simulink model "DCM_Pulse_Converter_Compare"  (R2019a)
settings: Solver=ode5  StartTime=0.0  StopTime=t_end  FixedStep=dt  RelTol=1e-3  EnableMultiTasking=on
values from neighbouring files (symbols this model uses):
  dt = 1e-5    (= 1e-05)    [Experiment_1_DCM_Parameter.m]
  T_c = 0    [Experiment_1_DCM_Parameter.m]
  T_CON = 0    [Experiment_1_DCM_Parameter.m]
  U_EN = 220    [Experiment_1_DCM_Parameter.m]
  V_CON = 0    [Experiment_1_DCM_Parameter.m]
libraries: simulink x1, powerlib x1
settings Model: Creator=BinLi  LastModifiedBy=Praktikum
settings DataIOCC: LimitDataPoints=on  SaveFormat=Array  SignalLoggingSaveFormat=ModelDataLogs  ReturnWorkspaceOutputs=off
settings OptimizationCC: ExpressionDepthLimit=2147483647  LifeSpan=inf
settings DebuggingCC: UnderspecifiedInitializationDetection=Classic  MergeDetectMultiDrivingBlocksExec=none  SolverPrmCheckMsg=warning  FcnCallInpInsideContextMsg=warning  StateNameClashWarn=warning  SFUnexpectedBacktrackingDiag=warning  SFNoUnconditionalDefaultTransitionDiag=warning  SFExecutionAtInitializationDiag=none  ArithmeticOperatorsInVariantConditions=warning
settings HardwareCC: ProdBitPerPointer=32  ProdBitPerSizeT=32  ProdBitPerPtrDiffT=32  ProdLargestAtomicFloat=None  ProdIntDivRoundTo=Undefined  ProdEndianess=Unspecified  ProdWordSize=32  ProdHWDeviceType=32-bit Generic
settings ModelReferenceCC: PropagateSignalLabelsOutOfModel=off
settings SFSimCC: SimUseLocalCustomCode=off  SimParseCustomCode=off
settings RTWCC: RTWUseLocalCustomCode=off
settings CodeAppCC: StateflowObjectComments=on
settings GRTTargetCC: TargetLangStandard=C89/C90 (ANSI)  CombineOutputUpdateFcns=off  GRTInterface=on
settings ConfigComp: CovMetricSettings=dw  CovSaveCumulativeToWorkspaceVar=on  CovSaveSingleToWorkspaceVar=on  CovExternalEMLEnable=off  CovSFcnEnable=off
settings SimscapeCC: SimscapeNormalizeSystem=off

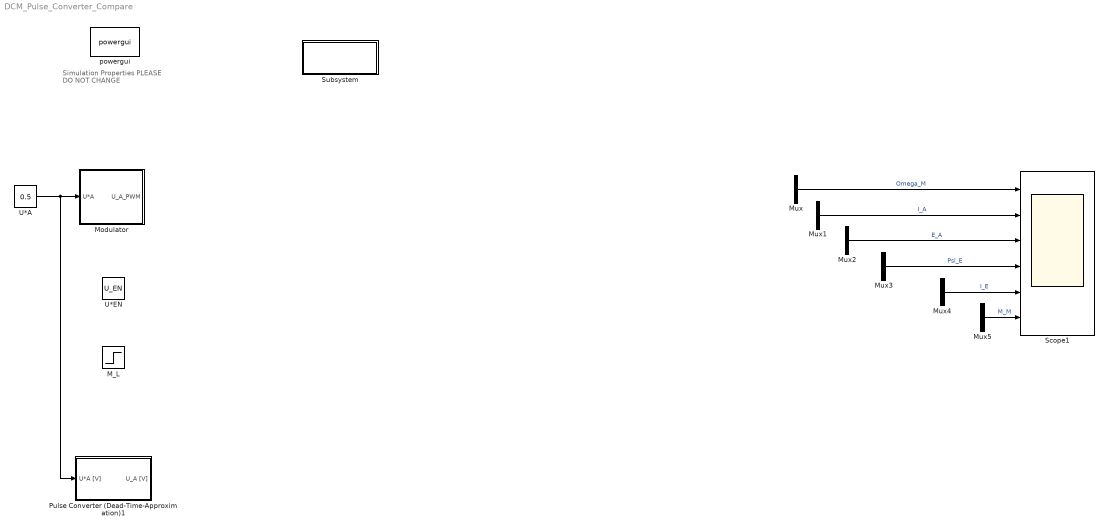
== system DCM_Pulse_Converter_Compare ==
  note: Simulation Properties
      | PLEASE DO NOT CHANGE
  M_L : Step  After=0.5  SampleTime=0
  Modulator : Subsystem
  Mux{,1..5} (6 alike) : Mux  Inputs=2
  Pulse Converter (Dead-Time-Approximation)1 : Subsystem
  Scope1 : Scope  NumInputPorts=6
  Subsystem : Subsystem
      settings: OpenFcn=Experiment_1_DCM_Parameter
      mask Display: disp('Initialize\n (doppelklicken)')
  U*A : Constant  Value=0.5
  U*EN : Constant  Value=U_EN
  powergui : powerlib/powergui  Priority=1  SimulationMode=Discrete  SampleTime=dt  frequency=60  Iterations=50  frequencyindice=0  Pbase=100e6  ErrMax=1e-4  UnitsV=kV  UnitsW=MW  buscounter=0  FunctionMessages=off  echomessages=off  EnableUseOfTLC=off  CurrentSourceSwitches=off  DisableSnubberDevices=off  DisableRonSwitches=off  DisableVfSwitches=off  DisplayEquations=off  AutomaticDiscreteSolvers=off  SolverType=Tustin  Interpol=off  ExternalGateDelay=off  methode=off  Ts=0  x0status=blocks  SPID=off  SwTol=0  HookPort=off  NonlinearTolerance=1e-4  nMaxIteration=100  ContinueOnMaxIteration=off  RestoreLinks=warning  ResistiveCurrentMeasurement=off  Frange=[0:2:500]  Ylog=off  Xlog=on  ShowGrid=off  save=off  variable=ZData  structure=0  ZoomFFT=off  StartTime=0.0  cycles=1  DisplayStyle=1  fundamental=60  FreqAxis=off  MaxFrequency=1000  frequencyindicesteady=1  RmsSteady=1  display=off
  wires:
  U*A/1 -> Modulator/1(U*A), Pulse Converter (Dead-Time-Approximation)1/1(U*A [V])
  Mux/1 -> Scope1/1  "Omega_M"
  Mux1/1 -> Scope1/2  "I_A"
  Mux2/1 -> Scope1/3  "E_A"
  Mux3/1 -> Scope1/4  "Psi_E"
  Mux4/1 -> Scope1/5  "I_E"
  Mux5/1 -> Scope1/6  "M_M"

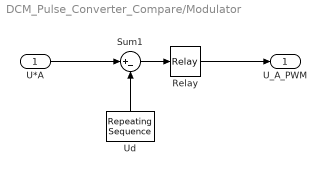
== system DCM_Pulse_Converter_Compare/Modulator ==
  U*A : Inport
  Relay : Relay  OnSwitchValue=1e-4  OffSwitchValue=-1e-4
  Sum1 : Sum  Inputs=|+-
  Ud : simulink/Sources/Repeating Sequence  rep_seq_t="[0 T_c/2  T_c]"  rep_seq_y=[1 -1 1]
  U_A_PWM : Outport
  wires:
  Ud/1 -> Sum1/2
  Sum1/1 -> Relay/1
  Relay/1 -> U_A_PWM/1
  U*A/1 -> Sum1/1

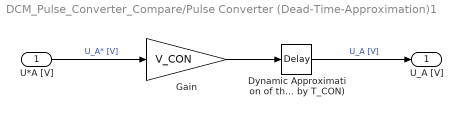
== system DCM_Pulse_Converter_Compare/Pulse Converter (Dead-Time-Approximation)1 ==
  U*A [V] : Inport
  Dynamic Approximation of the 2-level-converter (Delay by T_CON) : TransportDelay  DelayTime=T_CON
  Gain : Gain  Gain=V_CON
  U_A [V] : Outport
  wires:
  Dynamic Approximation of the 2-level-converter (Delay by T_CON)/1 -> U_A [V]/1  "U_A [V]"
  U*A [V]/1 -> Gain/1  "U_A* [V]"
  Gain/1 -> Dynamic Approximation of the 2-level-converter (Delay by T_CON)/1

== system DCM_Pulse_Converter_Compare/Subsystem ==
